simulink model "ex2_2"  (R2022a)
settings: Solver=VariableStepAuto  StartTime=0.0  StopTime=30  RelTol=1e-3
undefined symbols (not defined in the file): fdesignblkfcn, gcbh
libraries: dspfdesign x4, vrlib x1
settings Model: Creator=jeklu  LastModifiedBy=jeklu

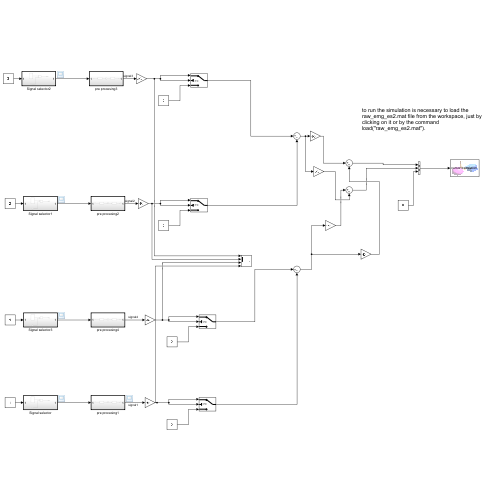
[thumbnail: Simulink's stored preview of the top-level diagram]
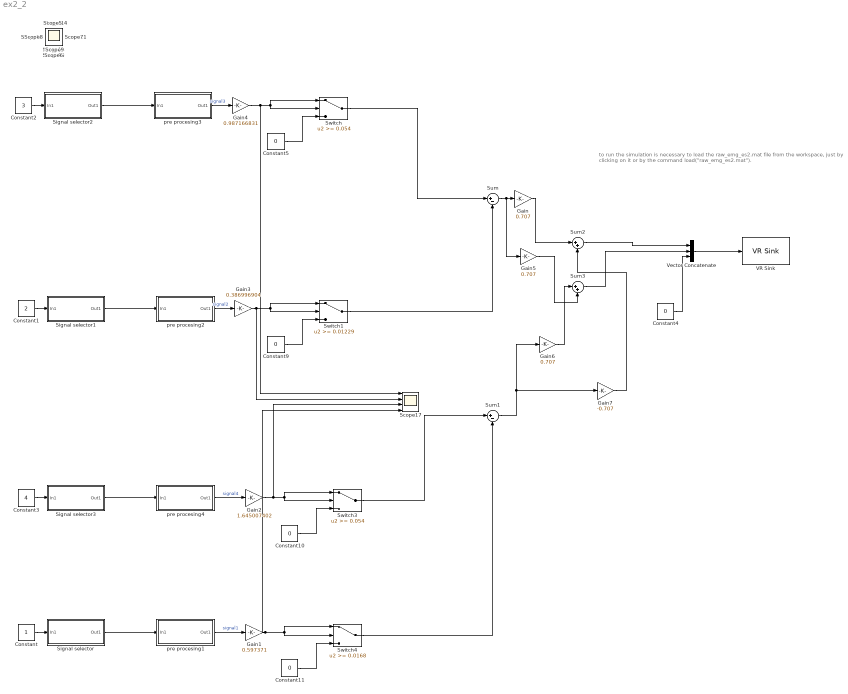
== system ex2_2 ==
  note: to run the simulation is necessary to load the raw_emg_es2.mat file from the workspace, just by clicking on it or by the command load("raw_emg_es2.mat").
  Constant : Constant  OutDataTypeStr=int8
  Constant1 : Constant  Value=2  OutDataTypeStr=int8
  Constant{4..5,9..11} (5 alike) : Constant  Value=0
  Constant2 : Constant  Value=3  OutDataTypeStr=int8
  Constant3 : Constant  Value=4  OutDataTypeStr=int8
  Gain : Gain  Gain=0.707
  Gain1 : Gain  Gain=0.597371
  Gain2 : Gain  Gain=1.645007402
  Gain3 : Gain  Gain=0.386996904
  Gain4 : Gain  Gain=0.987166831
  Gain5 : Gain  Gain=0.707
  Gain6 : Gain  Gain=0.707
  Gain7 : Gain  Gain=-0.707
  Scope17 : Scope  NumInputPorts=4
  Signal selector : Subsystem  TreatAsAtomicUnit=on
  Signal selector1 : Subsystem  TreatAsAtomicUnit=on
  Signal selector2 : Subsystem  TreatAsAtomicUnit=on
  Signal selector3 : Subsystem  TreatAsAtomicUnit=on
  Sum : Sum  Inputs=|+-
  Sum1 : Sum  Inputs=|+-
  Sum2 : Sum  Inputs=|++
  Sum3 : Sum  Inputs=|++
  Switch : Switch  Threshold=0.054  ZeroCross=off  SaturateOnIntegerOverflow=off  InputSameDT=off
  Switch1 : Switch  Threshold=0.01229  ZeroCross=off  SaturateOnIntegerOverflow=off  InputSameDT=off
  Switch3 : Switch  Threshold=0.054  ZeroCross=off  SaturateOnIntegerOverflow=off  InputSameDT=off
  Switch4 : Switch  Threshold=0.0168  ZeroCross=off  SaturateOnIntegerOverflow=off  InputSameDT=off
  VR Sink : vrlib/VR Sink  InstantiateOnLoad=on  SampleTime=0.1  ViewEnable=on  RemoteChange=off  RemoteView=off  FieldsWritten=cursor.translation.3.1.1.double  WorldFileName=8_palline_color.wrl  AutoView=off  VideoDimensions=[]  AllowVariableSize=off
  Vector Concatenate : Concatenate  NumInputs=3
  pre procesing1 : Subsystem  TreatAsAtomicUnit=on
  pre procesing2 : Subsystem  TreatAsAtomicUnit=on
  pre procesing3 : Subsystem  TreatAsAtomicUnit=on
  pre procesing4 : Subsystem  TreatAsAtomicUnit=on
  Scope{,1..15} (16 alike) : Scope
  wires:
  Constant/1 -> Signal selector/1(In1)
  Constant1/1 -> Signal selector1/1(In1)
  Constant3/1 -> Signal selector3/1(In1)
  Constant2/1 -> Signal selector2/1(In1)
  pre procesing3/1(Out1) -> Gain4/1  "signal3"
  pre procesing2/1(Out1) -> Gain3/1  "signal2"
  pre procesing1/1(Out1) -> Gain1/1  "signal1"
  pre procesing4/1(Out1) -> Gain2/1  "signal4"
  Signal selector/1(Out1) -> pre procesing1/1(In1)
  Signal selector3/1(Out1) -> pre procesing4/1(In1)
  Signal selector2/1(Out1) -> pre procesing3/1(In1)
  Signal selector1/1(Out1) -> pre procesing2/1(In1)
  Vector Concatenate/1 -> VR Sink/1
  Constant4/1 -> Vector Concatenate/3
  Switch/1 -> Sum/1
  Gain4/1 -> Scope17/1, Switch/2, Switch/1
  Constant5/1 -> Switch/3
  Switch1/1 -> Sum/2
  Constant9/1 -> Switch1/3
  Gain3/1 -> Scope17/2, Switch1/2, Switch1/1
  Constant10/1 -> Switch3/3
  Gain2/1 -> Switch3/1, Switch3/2, Scope17/3
  Constant11/1 -> Switch4/3
  Gain1/1 -> Switch4/2, Switch4/1, Scope17/4
  Switch3/1 -> Sum1/1
  Switch4/1 -> Sum1/2
  Sum/1 -> Gain5/1, Gain/1
  Sum2/1 -> Vector Concatenate/1
  Sum1/1 -> Gain7/1, Gain6/1
  Gain/1 -> Sum2/1
  Gain5/1 -> Sum3/2
  Gain6/1 -> Sum3/1
  Gain7/1 -> Sum2/2
  Sum3/1 -> Vector Concatenate/2

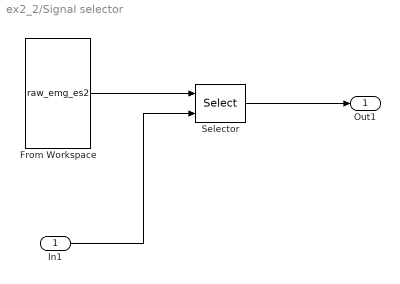
== system ex2_2/Signal selector ==
  In1 : Inport
  From Workspace : FromWorkspace  VariableName=raw_emg_es2
  Selector : Selector  InputPortWidth=4  IndexOptions=Starting index (port)  Indices=[1 3]  OutputSizes=1  RuntimeRangeChecks=on
  Out1 : Outport
  wires:
  Selector/1 -> Out1/1
  From Workspace/1 -> Selector/1
  In1/1 -> Selector/2

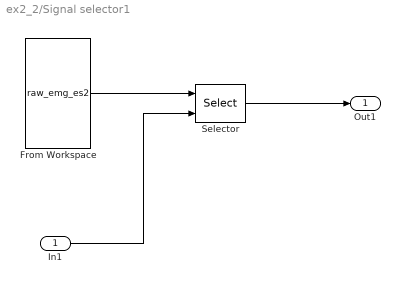
== system ex2_2/Signal selector1 ==
  In1 : Inport
  From Workspace : FromWorkspace  VariableName=raw_emg_es2
  Selector : Selector  InputPortWidth=4  IndexOptions=Starting index (port)  Indices=[1 3]  OutputSizes=1  RuntimeRangeChecks=on
  Out1 : Outport
  wires:
  Selector/1 -> Out1/1
  From Workspace/1 -> Selector/1
  In1/1 -> Selector/2

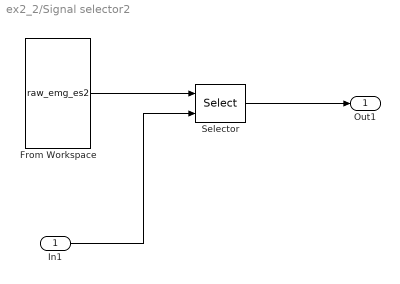
== system ex2_2/Signal selector2 ==
  In1 : Inport
  From Workspace : FromWorkspace  VariableName=raw_emg_es2
  Selector : Selector  InputPortWidth=4  IndexOptions=Starting index (port)  Indices=[1 3]  OutputSizes=1  RuntimeRangeChecks=on
  Out1 : Outport
  wires:
  Selector/1 -> Out1/1
  From Workspace/1 -> Selector/1
  In1/1 -> Selector/2

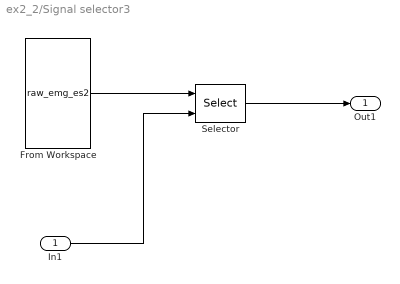
== system ex2_2/Signal selector3 ==
  In1 : Inport
  From Workspace : FromWorkspace  VariableName=raw_emg_es2
  Selector : Selector  InputPortWidth=4  IndexOptions=Starting index (port)  Indices=[1 3]  OutputSizes=1  RuntimeRangeChecks=on
  Out1 : Outport
  wires:
  Selector/1 -> Out1/1
  From Workspace/1 -> Selector/1
  In1/1 -> Selector/2

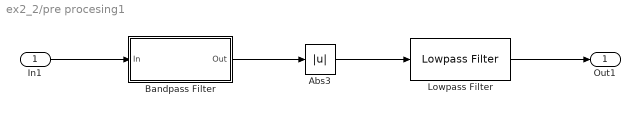
== system ex2_2/pre procesing1 ==
  In1 : Inport
  Abs3 : Abs  SaturateOnIntegerOverflow=off
  Bandpass Filter : Subsystem  DialogController=fdesignblkfcn  InitFcn=fdesignblkfcn(gcbh, {'InitFcn'});  mask(Bandpass Filter){}
      mask help: Design a bandpass filter
      settings: CopyFcn=fdesignblkfcn(gcbh, {'CopyFcn'});
      mask Help: helpview(mapfilelocation('dsp'), 'dspbandpassfilter');
      mask Display: disp('Bandpass');
  Lowpass Filter : dspfdesign/Lowpass Filter  FilterType=FIR  DesignForMinimumOrder=off  FilterOrder=10  PassbandFrequency=5  StopbandFrequency=6  PassbandRipple=0.1  StopbandAttenuation=80  InheritSampleRate=off  SampleRate=1000  SimulateUsing=Interpreted execution  roundingMode=Floor  coeffsDataTypeStr=fixdt(1,16)
  Out1 : Outport
  wires:
  Bandpass Filter/1(Out) -> Abs3/1
  In1/1 -> Bandpass Filter/1(In)
  Abs3/1 -> Lowpass Filter/1
  Lowpass Filter/1 -> Out1/1

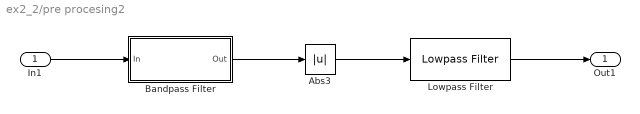
== system ex2_2/pre procesing2 ==
  In1 : Inport
  Abs3 : Abs  SaturateOnIntegerOverflow=off
  Bandpass Filter : Subsystem  DialogController=fdesignblkfcn  InitFcn=fdesignblkfcn(gcbh, {'InitFcn'});  mask(Bandpass Filter){}
      mask help: Design a bandpass filter
      settings: CopyFcn=fdesignblkfcn(gcbh, {'CopyFcn'});
      mask Help: helpview(mapfilelocation('dsp'), 'dspbandpassfilter');
      mask Display: disp('Bandpass');
  Lowpass Filter : dspfdesign/Lowpass Filter  FilterType=FIR  DesignForMinimumOrder=off  FilterOrder=10  PassbandFrequency=5  StopbandFrequency=6  PassbandRipple=0.1  StopbandAttenuation=80  InheritSampleRate=off  SampleRate=1000  SimulateUsing=Interpreted execution  roundingMode=Floor  coeffsDataTypeStr=fixdt(1,16)
  Out1 : Outport
  wires:
  Bandpass Filter/1(Out) -> Abs3/1
  In1/1 -> Bandpass Filter/1(In)
  Abs3/1 -> Lowpass Filter/1
  Lowpass Filter/1 -> Out1/1

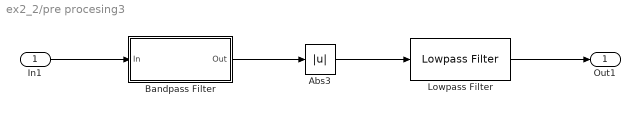
== system ex2_2/pre procesing3 ==
  In1 : Inport
  Abs3 : Abs  SaturateOnIntegerOverflow=off
  Bandpass Filter : Subsystem  DialogController=fdesignblkfcn  InitFcn=fdesignblkfcn(gcbh, {'InitFcn'});  mask(Bandpass Filter){}
      mask help: Design a bandpass filter
      settings: CopyFcn=fdesignblkfcn(gcbh, {'CopyFcn'});
      mask Help: helpview(mapfilelocation('dsp'), 'dspbandpassfilter');
      mask Display: disp('Bandpass');
  Lowpass Filter : dspfdesign/Lowpass Filter  FilterType=FIR  DesignForMinimumOrder=off  FilterOrder=10  PassbandFrequency=5  StopbandFrequency=6  PassbandRipple=0.1  StopbandAttenuation=80  InheritSampleRate=off  SampleRate=1000  SimulateUsing=Interpreted execution  roundingMode=Floor  coeffsDataTypeStr=fixdt(1,16)
  Out1 : Outport
  wires:
  Bandpass Filter/1(Out) -> Abs3/1
  In1/1 -> Bandpass Filter/1(In)
  Abs3/1 -> Lowpass Filter/1
  Lowpass Filter/1 -> Out1/1

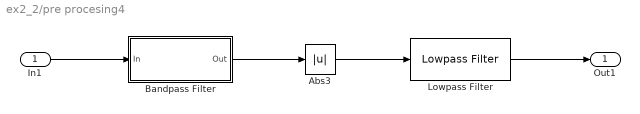
== system ex2_2/pre procesing4 ==
  In1 : Inport
  Abs3 : Abs  SaturateOnIntegerOverflow=off
  Bandpass Filter : Subsystem  DialogController=fdesignblkfcn  InitFcn=fdesignblkfcn(gcbh, {'InitFcn'});  mask(Bandpass Filter){}
      mask help: Design a bandpass filter
      settings: CopyFcn=fdesignblkfcn(gcbh, {'CopyFcn'});
      mask Help: helpview(mapfilelocation('dsp'), 'dspbandpassfilter');
      mask Display: disp('Bandpass');
  Lowpass Filter : dspfdesign/Lowpass Filter  FilterType=FIR  DesignForMinimumOrder=off  FilterOrder=10  PassbandFrequency=5  StopbandFrequency=6  PassbandRipple=0.1  StopbandAttenuation=80  InheritSampleRate=off  SampleRate=1000  SimulateUsing=Interpreted execution  roundingMode=Floor  coeffsDataTypeStr=fixdt(1,16)
  Out1 : Outport
  wires:
  Bandpass Filter/1(Out) -> Abs3/1
  In1/1 -> Bandpass Filter/1(In)
  Abs3/1 -> Lowpass Filter/1
  Lowpass Filter/1 -> Out1/1

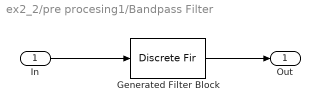
== system ex2_2/pre procesing1/Bandpass Filter ==
  In : Inport
  Generated Filter Block : DiscreteFir  Tag=BlockMethodSubSystem  Coefficients=[0.0118271107278146211 0.00749421447574264571 -0.0610262833618276795 -0.00697141743860507472 -0.0116983880847790316 -0.00563959661055920408 -0.00154341643986332169 -0.00513754171063308344 0.00172228706187026984 -0.00526958376803667288 0.00359194610790952631 -0.00514151489691697453 0.00474817145150627142 -0.00433598087152893726 0.00511197423488456149 -0.00281615651890120607 0.00471362178833440847 -0.000884551681865184997 0.00379617769311047654 0.000962848608355189447 0.00276101841748683727 0.00217953760066745376 0.00201440099357166631 0.00236555191439876116 0.0017951524066038096 0.00141965583780424105 0.0020985880028889666 -0.000410709871371749428 0.00264892030593250147 -0.00260011965921140478 0.00302215798560306111 -0.00450794219530739528 0.00283156413594070787 -0.00558916491529372686 0.00188583503180307557 -0.00557248571572052306 0.000292203201136945689 -0.00454166538989120034 -0.00153123569293347789 -0.00290656256385710566 -0.00298837227713725411 -0.00123582962926981261 -0.00351434986432584045 -4.92425425002664778e-05 -0.00278629972078519271 0.000362431324371223051 -0.000859790375592845162 4.5538858277097793e-05 0.00181113997287808367 -0.000636067330199022239 0.00448524325969081473 -0.00117465125005462834 0.0063831720375287478 -0.00112244535320554827 0.00693805469647473198 -0.000287698294534470946 0.00597506593640754168 0.00114347587240745262 0.00379154014009846834 0.0026525143849507422 0.00106730249876277414 0.0035698062181322137 -0.00140352762396881185 0.00331993911350809577 -0.00293956759205080218 0.00166764782777376595 -0.00322436690262694085 -0.00112597611597016522 -0.00242506730787882653 -0.0043749623011553971 -0.00106058404383880308 -0.00710426121963035964 0.000135937082787558611 -0.00842264322081914124 0.000622455362958887503 -0.00779254229350853297 0.000101781023988114494 -0.00524409663420731705 -0.00102497087743313141 -0.0014337505835135629 -0.00233931575929311603 0.00261666745863818129 -0.00274178754521887599 0.00575284402411575628 -0.00187627507344668119 0.00716367863413789642 0.000488603187998676953 0.00657375227120330936 0.00397196831299415163 0.00438243971482460068 0.00744629810190213046 0.00148133478353088444 0.00968581695133780875 -0.00105968846398337888 0.00976044500007753647 -0.002411259358405807 0.00722142862482566712 -0.00227842939601705314 0.00237632127158438284 -0.0010312494154450895 -0.00362396782292390748 0.00042445260458756867 -0.00912615321763714585 0.00100768652351161388 -0.01251791509973991 -8.3073931949456648e-05 -0.01277506974576007 -0.00296463690336018666 -0.00979904358787195631 -0.00689021760160115574 -0.00447874931474320261 -0.0104099638934214353 0.00156559383624149564 -0.0118341918315854888 0.00652138748948258382 -0.00983855022393172185 0.00901450099974570457 -0.00404503888266741739 0.00858744454369512328 0.0046647480902971359 0.00588627913719553999 0.0142212352936126572 0.00247719174881328363 0.0218568610073119479 0.000284751276763566897 0.0249113149306009231 0.000798255704818454678 0.0217050789571666715 0.00434485112370316864 0.0121771979949330672 0.00976045660276175786 -0.00188161452234936384 0.0144764327260983958 -0.0171520620746796505 0.0150843353936123224 -0.0296385008929091337 0.00836912193791909675 -0.0357558888299704739 -0.00758761695197321395 -0.0333867705962057962 -0.0326783507431195677 -0.0225858736803771117 -0.0643641534905359525 -0.00570504529169045191 -0.0979964325310505591 0.0132053087046869102 -0.127909324620181619 0.0293693909135900461 -0.14851337210877999 0.0386616039021836361 0.844118884495555943 0.0386616039021836361 -0.14851337210877999 0.0293693909135900461 -0.127909324620181619 0.0132053087046869102 -0.0979964325310505591 -0.00570504529169045191 -0.0643641534905359525 -0.0225858736803771117 -0.0326783507431195677 -0.0333867705962057962 -0.00758761695197321395 -0.0357558888299704739 0.00836912193791909675 -0.0296385008929091337 0.0150843353936123224 -0.0171520620746796505 0.0144764327260983958 -0.00188161452234936384 0.00976045660276175786 0.0121771979949330672 ...(+3018 chars)]  InputProcessing=Columns as channels (frame based)
  Out : Outport  VectorParamsAs1DForOutWhenUnconnected=off
  wires:
  In/1 -> Generated Filter Block/1
  Generated Filter Block/1 -> Out/1

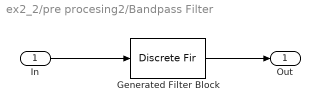
== system ex2_2/pre procesing2/Bandpass Filter ==
  In : Inport
  Generated Filter Block : DiscreteFir  Tag=BlockMethodSubSystem  Coefficients=[0.0118271107278146211 0.00749421447574264571 -0.0610262833618276795 -0.00697141743860507472 -0.0116983880847790316 -0.00563959661055920408 -0.00154341643986332169 -0.00513754171063308344 0.00172228706187026984 -0.00526958376803667288 0.00359194610790952631 -0.00514151489691697453 0.00474817145150627142 -0.00433598087152893726 0.00511197423488456149 -0.00281615651890120607 0.00471362178833440847 -0.000884551681865184997 0.00379617769311047654 0.000962848608355189447 0.00276101841748683727 0.00217953760066745376 0.00201440099357166631 0.00236555191439876116 0.0017951524066038096 0.00141965583780424105 0.0020985880028889666 -0.000410709871371749428 0.00264892030593250147 -0.00260011965921140478 0.00302215798560306111 -0.00450794219530739528 0.00283156413594070787 -0.00558916491529372686 0.00188583503180307557 -0.00557248571572052306 0.000292203201136945689 -0.00454166538989120034 -0.00153123569293347789 -0.00290656256385710566 -0.00298837227713725411 -0.00123582962926981261 -0.00351434986432584045 -4.92425425002664778e-05 -0.00278629972078519271 0.000362431324371223051 -0.000859790375592845162 4.5538858277097793e-05 0.00181113997287808367 -0.000636067330199022239 0.00448524325969081473 -0.00117465125005462834 0.0063831720375287478 -0.00112244535320554827 0.00693805469647473198 -0.000287698294534470946 0.00597506593640754168 0.00114347587240745262 0.00379154014009846834 0.0026525143849507422 0.00106730249876277414 0.0035698062181322137 -0.00140352762396881185 0.00331993911350809577 -0.00293956759205080218 0.00166764782777376595 -0.00322436690262694085 -0.00112597611597016522 -0.00242506730787882653 -0.0043749623011553971 -0.00106058404383880308 -0.00710426121963035964 0.000135937082787558611 -0.00842264322081914124 0.000622455362958887503 -0.00779254229350853297 0.000101781023988114494 -0.00524409663420731705 -0.00102497087743313141 -0.0014337505835135629 -0.00233931575929311603 0.00261666745863818129 -0.00274178754521887599 0.00575284402411575628 -0.00187627507344668119 0.00716367863413789642 0.000488603187998676953 0.00657375227120330936 0.00397196831299415163 0.00438243971482460068 0.00744629810190213046 0.00148133478353088444 0.00968581695133780875 -0.00105968846398337888 0.00976044500007753647 -0.002411259358405807 0.00722142862482566712 -0.00227842939601705314 0.00237632127158438284 -0.0010312494154450895 -0.00362396782292390748 0.00042445260458756867 -0.00912615321763714585 0.00100768652351161388 -0.01251791509973991 -8.3073931949456648e-05 -0.01277506974576007 -0.00296463690336018666 -0.00979904358787195631 -0.00689021760160115574 -0.00447874931474320261 -0.0104099638934214353 0.00156559383624149564 -0.0118341918315854888 0.00652138748948258382 -0.00983855022393172185 0.00901450099974570457 -0.00404503888266741739 0.00858744454369512328 0.0046647480902971359 0.00588627913719553999 0.0142212352936126572 0.00247719174881328363 0.0218568610073119479 0.000284751276763566897 0.0249113149306009231 0.000798255704818454678 0.0217050789571666715 0.00434485112370316864 0.0121771979949330672 0.00976045660276175786 -0.00188161452234936384 0.0144764327260983958 -0.0171520620746796505 0.0150843353936123224 -0.0296385008929091337 0.00836912193791909675 -0.0357558888299704739 -0.00758761695197321395 -0.0333867705962057962 -0.0326783507431195677 -0.0225858736803771117 -0.0643641534905359525 -0.00570504529169045191 -0.0979964325310505591 0.0132053087046869102 -0.127909324620181619 0.0293693909135900461 -0.14851337210877999 0.0386616039021836361 0.844118884495555943 0.0386616039021836361 -0.14851337210877999 0.0293693909135900461 -0.127909324620181619 0.0132053087046869102 -0.0979964325310505591 -0.00570504529169045191 -0.0643641534905359525 -0.0225858736803771117 -0.0326783507431195677 -0.0333867705962057962 -0.00758761695197321395 -0.0357558888299704739 0.00836912193791909675 -0.0296385008929091337 0.0150843353936123224 -0.0171520620746796505 0.0144764327260983958 -0.00188161452234936384 0.00976045660276175786 0.0121771979949330672 ...(+3018 chars)]  InputProcessing=Columns as channels (frame based)
  Out : Outport  VectorParamsAs1DForOutWhenUnconnected=off
  wires:
  In/1 -> Generated Filter Block/1
  Generated Filter Block/1 -> Out/1

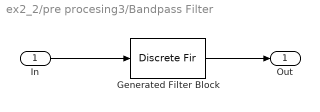
== system ex2_2/pre procesing3/Bandpass Filter ==
  In : Inport
  Generated Filter Block : DiscreteFir  Tag=BlockMethodSubSystem  Coefficients=[0.0118271107278146211 0.00749421447574264571 -0.0610262833618276795 -0.00697141743860507472 -0.0116983880847790316 -0.00563959661055920408 -0.00154341643986332169 -0.00513754171063308344 0.00172228706187026984 -0.00526958376803667288 0.00359194610790952631 -0.00514151489691697453 0.00474817145150627142 -0.00433598087152893726 0.00511197423488456149 -0.00281615651890120607 0.00471362178833440847 -0.000884551681865184997 0.00379617769311047654 0.000962848608355189447 0.00276101841748683727 0.00217953760066745376 0.00201440099357166631 0.00236555191439876116 0.0017951524066038096 0.00141965583780424105 0.0020985880028889666 -0.000410709871371749428 0.00264892030593250147 -0.00260011965921140478 0.00302215798560306111 -0.00450794219530739528 0.00283156413594070787 -0.00558916491529372686 0.00188583503180307557 -0.00557248571572052306 0.000292203201136945689 -0.00454166538989120034 -0.00153123569293347789 -0.00290656256385710566 -0.00298837227713725411 -0.00123582962926981261 -0.00351434986432584045 -4.92425425002664778e-05 -0.00278629972078519271 0.000362431324371223051 -0.000859790375592845162 4.5538858277097793e-05 0.00181113997287808367 -0.000636067330199022239 0.00448524325969081473 -0.00117465125005462834 0.0063831720375287478 -0.00112244535320554827 0.00693805469647473198 -0.000287698294534470946 0.00597506593640754168 0.00114347587240745262 0.00379154014009846834 0.0026525143849507422 0.00106730249876277414 0.0035698062181322137 -0.00140352762396881185 0.00331993911350809577 -0.00293956759205080218 0.00166764782777376595 -0.00322436690262694085 -0.00112597611597016522 -0.00242506730787882653 -0.0043749623011553971 -0.00106058404383880308 -0.00710426121963035964 0.000135937082787558611 -0.00842264322081914124 0.000622455362958887503 -0.00779254229350853297 0.000101781023988114494 -0.00524409663420731705 -0.00102497087743313141 -0.0014337505835135629 -0.00233931575929311603 0.00261666745863818129 -0.00274178754521887599 0.00575284402411575628 -0.00187627507344668119 0.00716367863413789642 0.000488603187998676953 0.00657375227120330936 0.00397196831299415163 0.00438243971482460068 0.00744629810190213046 0.00148133478353088444 0.00968581695133780875 -0.00105968846398337888 0.00976044500007753647 -0.002411259358405807 0.00722142862482566712 -0.00227842939601705314 0.00237632127158438284 -0.0010312494154450895 -0.00362396782292390748 0.00042445260458756867 -0.00912615321763714585 0.00100768652351161388 -0.01251791509973991 -8.3073931949456648e-05 -0.01277506974576007 -0.00296463690336018666 -0.00979904358787195631 -0.00689021760160115574 -0.00447874931474320261 -0.0104099638934214353 0.00156559383624149564 -0.0118341918315854888 0.00652138748948258382 -0.00983855022393172185 0.00901450099974570457 -0.00404503888266741739 0.00858744454369512328 0.0046647480902971359 0.00588627913719553999 0.0142212352936126572 0.00247719174881328363 0.0218568610073119479 0.000284751276763566897 0.0249113149306009231 0.000798255704818454678 0.0217050789571666715 0.00434485112370316864 0.0121771979949330672 0.00976045660276175786 -0.00188161452234936384 0.0144764327260983958 -0.0171520620746796505 0.0150843353936123224 -0.0296385008929091337 0.00836912193791909675 -0.0357558888299704739 -0.00758761695197321395 -0.0333867705962057962 -0.0326783507431195677 -0.0225858736803771117 -0.0643641534905359525 -0.00570504529169045191 -0.0979964325310505591 0.0132053087046869102 -0.127909324620181619 0.0293693909135900461 -0.14851337210877999 0.0386616039021836361 0.844118884495555943 0.0386616039021836361 -0.14851337210877999 0.0293693909135900461 -0.127909324620181619 0.0132053087046869102 -0.0979964325310505591 -0.00570504529169045191 -0.0643641534905359525 -0.0225858736803771117 -0.0326783507431195677 -0.0333867705962057962 -0.00758761695197321395 -0.0357558888299704739 0.00836912193791909675 -0.0296385008929091337 0.0150843353936123224 -0.0171520620746796505 0.0144764327260983958 -0.00188161452234936384 0.00976045660276175786 0.0121771979949330672 ...(+3018 chars)]  InputProcessing=Columns as channels (frame based)
  Out : Outport  VectorParamsAs1DForOutWhenUnconnected=off
  wires:
  In/1 -> Generated Filter Block/1
  Generated Filter Block/1 -> Out/1

== system ex2_2/pre procesing4/Bandpass Filter ==
  In : Inport
  Generated Filter Block : DiscreteFir  Tag=BlockMethodSubSystem  Coefficients=[0.0118271107278146211 0.00749421447574264571 -0.0610262833618276795 -0.00697141743860507472 -0.0116983880847790316 -0.00563959661055920408 -0.00154341643986332169 -0.00513754171063308344 0.00172228706187026984 -0.00526958376803667288 0.00359194610790952631 -0.00514151489691697453 0.00474817145150627142 -0.00433598087152893726 0.00511197423488456149 -0.00281615651890120607 0.00471362178833440847 -0.000884551681865184997 0.00379617769311047654 0.000962848608355189447 0.00276101841748683727 0.00217953760066745376 0.00201440099357166631 0.00236555191439876116 0.0017951524066038096 0.00141965583780424105 0.0020985880028889666 -0.000410709871371749428 0.00264892030593250147 -0.00260011965921140478 0.00302215798560306111 -0.00450794219530739528 0.00283156413594070787 -0.00558916491529372686 0.00188583503180307557 -0.00557248571572052306 0.000292203201136945689 -0.00454166538989120034 -0.00153123569293347789 -0.00290656256385710566 -0.00298837227713725411 -0.00123582962926981261 -0.00351434986432584045 -4.92425425002664778e-05 -0.00278629972078519271 0.000362431324371223051 -0.000859790375592845162 4.5538858277097793e-05 0.00181113997287808367 -0.000636067330199022239 0.00448524325969081473 -0.00117465125005462834 0.0063831720375287478 -0.00112244535320554827 0.00693805469647473198 -0.000287698294534470946 0.00597506593640754168 0.00114347587240745262 0.00379154014009846834 0.0026525143849507422 0.00106730249876277414 0.0035698062181322137 -0.00140352762396881185 0.00331993911350809577 -0.00293956759205080218 0.00166764782777376595 -0.00322436690262694085 -0.00112597611597016522 -0.00242506730787882653 -0.0043749623011553971 -0.00106058404383880308 -0.00710426121963035964 0.000135937082787558611 -0.00842264322081914124 0.000622455362958887503 -0.00779254229350853297 0.000101781023988114494 -0.00524409663420731705 -0.00102497087743313141 -0.0014337505835135629 -0.00233931575929311603 0.00261666745863818129 -0.00274178754521887599 0.00575284402411575628 -0.00187627507344668119 0.00716367863413789642 0.000488603187998676953 0.00657375227120330936 0.00397196831299415163 0.00438243971482460068 0.00744629810190213046 0.00148133478353088444 0.00968581695133780875 -0.00105968846398337888 0.00976044500007753647 -0.002411259358405807 0.00722142862482566712 -0.00227842939601705314 0.00237632127158438284 -0.0010312494154450895 -0.00362396782292390748 0.00042445260458756867 -0.00912615321763714585 0.00100768652351161388 -0.01251791509973991 -8.3073931949456648e-05 -0.01277506974576007 -0.00296463690336018666 -0.00979904358787195631 -0.00689021760160115574 -0.00447874931474320261 -0.0104099638934214353 0.00156559383624149564 -0.0118341918315854888 0.00652138748948258382 -0.00983855022393172185 0.00901450099974570457 -0.00404503888266741739 0.00858744454369512328 0.0046647480902971359 0.00588627913719553999 0.0142212352936126572 0.00247719174881328363 0.0218568610073119479 0.000284751276763566897 0.0249113149306009231 0.000798255704818454678 0.0217050789571666715 0.00434485112370316864 0.0121771979949330672 0.00976045660276175786 -0.00188161452234936384 0.0144764327260983958 -0.0171520620746796505 0.0150843353936123224 -0.0296385008929091337 0.00836912193791909675 -0.0357558888299704739 -0.00758761695197321395 -0.0333867705962057962 -0.0326783507431195677 -0.0225858736803771117 -0.0643641534905359525 -0.00570504529169045191 -0.0979964325310505591 0.0132053087046869102 -0.127909324620181619 0.0293693909135900461 -0.14851337210877999 0.0386616039021836361 0.844118884495555943 0.0386616039021836361 -0.14851337210877999 0.0293693909135900461 -0.127909324620181619 0.0132053087046869102 -0.0979964325310505591 -0.00570504529169045191 -0.0643641534905359525 -0.0225858736803771117 -0.0326783507431195677 -0.0333867705962057962 -0.00758761695197321395 -0.0357558888299704739 0.00836912193791909675 -0.0296385008929091337 0.0150843353936123224 -0.0171520620746796505 0.0144764327260983958 -0.00188161452234936384 0.00976045660276175786 0.0121771979949330672 ...(+3018 chars)]  InputProcessing=Columns as channels (frame based)
  Out : Outport  VectorParamsAs1DForOutWhenUnconnected=off
  wires:
  In/1 -> Generated Filter Block/1
  Generated Filter Block/1 -> Out/1
